simulink model "Lab4"  (R2022b)
settings: Solver=VariableStepAuto  StartTime=0.0  StopTime=10.0  MaxStep=1e-3  RelTol=1e-3
libraries: simulink x7
settings Model: Creator=LOQ  LastModifiedBy=LOQ
settings OptimizationCC: ReuseModelBlockBuffer=on
settings RTWCC: GPUComputeCapability=5.0
settings ConfigComp: CovBoundaryAbsTol=1.0e-5

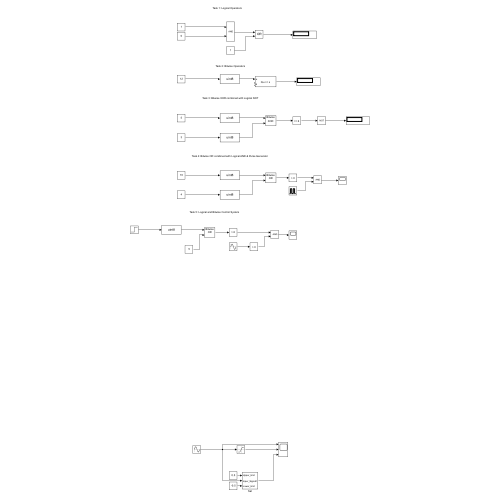
[thumbnail: Simulink's stored preview of the top-level diagram]
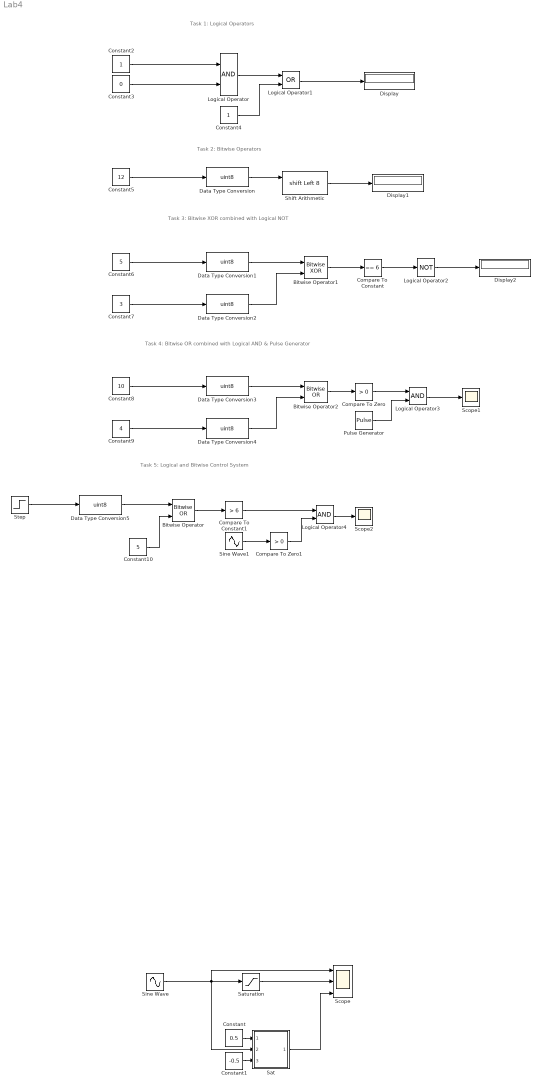
== system Lab4 ==
  note: Task 5: Logical and Bitwise Control System
  note: Task 4: Bitwise OR combined with Logical AND & Pulse Generator
  note: Task 3: Bitwise XOR combined with Logical NOT
  note: Task 2: Bitwise Operators
  note: Task 1: Logical Operators
  Bitwise Operator : simulink/Logic and Bit Operations/Bitwise Operator  logicop=OR  UseBitMask=off  NumInputPorts=2  BitMask=bin2dec('11011001')  BitMaskRealWorld=Stored Integer
  Bitwise Operator1 : simulink/Logic and Bit Operations/Bitwise Operator  logicop=XOR  UseBitMask=off  NumInputPorts=2  BitMask=bin2dec('11011001')  BitMaskRealWorld=Stored Integer
  Bitwise Operator2 : simulink/Logic and Bit Operations/Bitwise Operator  logicop=OR  UseBitMask=off  NumInputPorts=2  BitMask=bin2dec('11011001')  BitMaskRealWorld=Stored Integer
  Compare To Constant : simulink/Logic and Bit Operations/Compare To Constant  relop===  const=6  OutDataTypeStr=boolean
  Compare To Constant1 : simulink/Logic and Bit Operations/Compare To Constant  relop=>  const=6  OutDataTypeStr=boolean
  Compare To Zero : simulink/Logic and Bit Operations/Compare To Zero  relop=>  OutDataTypeStr=boolean
  Compare To Zero1 : simulink/Logic and Bit Operations/Compare To Zero  relop=>  OutDataTypeStr=boolean
  Constant : Constant  Value=0.5
  Constant1 : Constant  Value=-0.5
  Constant10 : Constant  Value=5  OutDataTypeStr=uint8
  Constant2 : Constant
  Constant3 : Constant  Value=0
  Constant4 : Constant
  Constant5 : Constant  Value=12
  Constant6 : Constant  Value=5
  Constant7 : Constant  Value=3
  Constant8 : Constant  Value=10
  Constant9 : Constant  Value=4
  Data Type Conversion{,1..5} (6 alike) : DataTypeConversion  OutDataTypeStr=uint8  SaturateOnIntegerOverflow=off  RndMeth=Floor
  Display : Display
  Display1 : Display
  Display2 : Display
  Logical Operator : Logic  AllPortsSameDT=off  OutDataTypeStr=boolean
  Logical Operator1 : Logic  Operator=OR  AllPortsSameDT=off  OutDataTypeStr=boolean
  Logical Operator2 : Logic  Operator=NOT  AllPortsSameDT=off  OutDataTypeStr=boolean
  Logical Operator3 : Logic  AllPortsSameDT=off  OutDataTypeStr=boolean
  Logical Operator4 : Logic  AllPortsSameDT=off  OutDataTypeStr=boolean
  Pulse Generator : DiscretePulseGenerator  PulseType=Time based  PulseWidth=50
  Sat : Subsystem
  Saturation : Saturate
  Scope : Scope  NumInputPorts=3
  Scope1 : Scope
  Scope2 : Scope
  Shift Arithmetic : ArithShift  BitShiftNumberSource=Input port  BitShiftNumber=8  BitShiftDirection=Left
      settings: InputPortMap=u0,p1
  Sine Wave : Sin  SampleTime=0
  Sine Wave1 : Sin  SampleTime=0
  Step : Step  Time=5  After=3  SampleTime=0
  wires:
  Sine Wave/1 -> Sat/2(Inpur_Signal), Scope/1, Saturation/1
  Saturation/1 -> Scope/2
  Constant/1 -> Sat/1(Upper_limit)
  Constant1/1 -> Sat/3(Lower_limit)
  Sat/1(Output) -> Scope/3
  Constant2/1 -> Logical Operator/1
  Constant3/1 -> Logical Operator/2
  Logical Operator/1 -> Logical Operator1/1
  Constant4/1 -> Logical Operator1/2
  Logical Operator1/1 -> Display/1
  Constant5/1 -> Data Type Conversion/1
  Data Type Conversion/1 -> Shift Arithmetic/1
  Constant6/1 -> Data Type Conversion1/1
  Constant7/1 -> Data Type Conversion2/1
  Data Type Conversion1/1 -> Bitwise Operator1/1
  Data Type Conversion2/1 -> Bitwise Operator1/2
  Bitwise Operator1/1 -> Compare To Constant/1
  Compare To Constant/1 -> Logical Operator2/1
  Logical Operator2/1 -> Display2/1
  Constant9/1 -> Data Type Conversion4/1
  Constant8/1 -> Data Type Conversion3/1
  Data Type Conversion4/1 -> Bitwise Operator2/2
  Data Type Conversion3/1 -> Bitwise Operator2/1
  Bitwise Operator2/1 -> Compare To Zero/1
  Compare To Zero/1 -> Logical Operator3/1
  Pulse Generator/1 -> Logical Operator3/2
  Logical Operator3/1 -> Scope1/1
  Shift Arithmetic/1 -> Display1/1
  Step/1 -> Data Type Conversion5/1
  Data Type Conversion5/1 -> Bitwise Operator/1
  Constant10/1 -> Bitwise Operator/2
  Bitwise Operator/1 -> Compare To Constant1/1
  Sine Wave1/1 -> Compare To Zero1/1
  Compare To Constant1/1 -> Logical Operator4/1
  Compare To Zero1/1 -> Logical Operator4/2
  Logical Operator4/1 -> Scope2/1

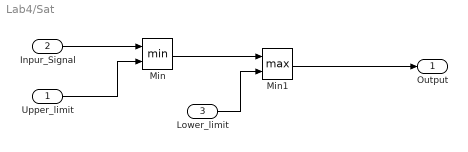
== system Lab4/Sat ==
  Upper_limit : Inport
  Inpur_Signal : Inport  Port=2
  Lower_limit : Inport  Port=3
  Min : MinMax  Inputs=2
  Min1 : MinMax  Function=max  Inputs=2
  Output : Outport
  wires:
  Min/1 -> Min1/1
  Lower_limit/1 -> Min1/2
  Upper_limit/1 -> Min/2
  Inpur_Signal/1 -> Min/1
  Min1/1 -> Output/1
